simulink model "attempt99999"  (R2026a)
settings: Solver=VariableStepAuto  StopTime=10
values from neighbouring files (symbols this model uses):
  I_x = 3770    [attempt999999.m]
  I_y = 730    [attempt999999.m]
  I_z = 4020    [attempt999999.m]
  omega_0 = 7.272 * 10^-5    (= 7.272e-05)    [attempt999999.m]
settings Model: Creator=syane  LastModifiedBy=syane

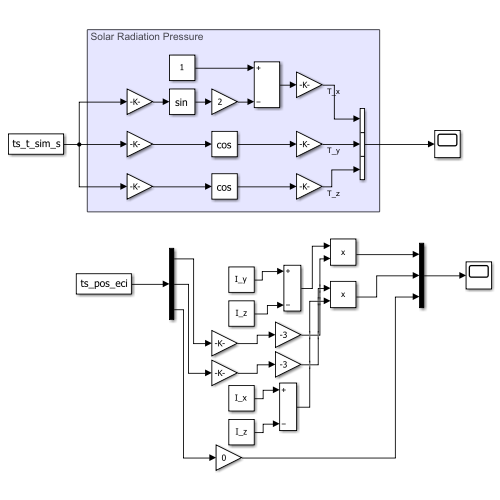
[thumbnail: Simulink's stored preview of the top-level diagram]
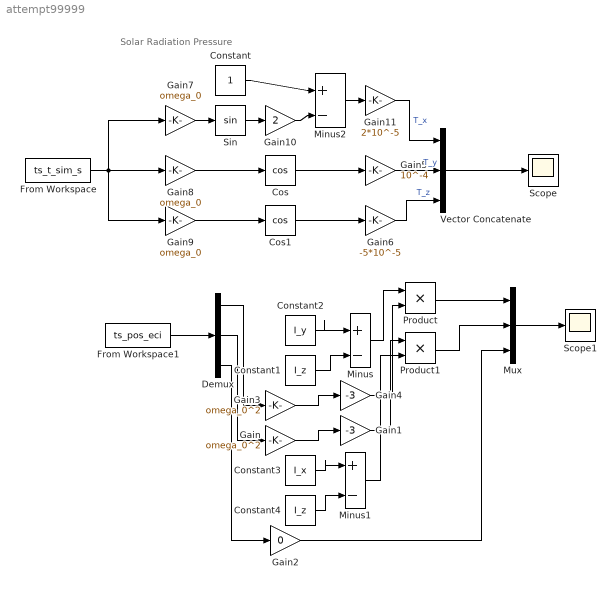
== system attempt99999 ==
  note: Solar Radiation Pressure
  Constant : Constant
  Constant1 : Constant  Value=I_z
  Constant2 : Constant  Value=I_y
  Constant3 : Constant  Value=I_x
  Constant4 : Constant  Value=I_z
  Cos : Trigonometry  Operator=cos
  Cos1 : Trigonometry  Operator=cos
  Demux : Demux  Outputs=3
  From Workspace : FromWorkspace  VariableName=ts_t_sim_s
  From Workspace1 : FromWorkspace  VariableName=ts_pos_eci
  Gain : Gain  Gain=omega_0^2
  Gain1 : Gain  Gain=-3
  Gain10 : Gain  Gain=2
  Gain11 : Gain  Gain=2*10^-5
  Gain2 : Gain  Gain=0
  Gain3 : Gain  Gain=omega_0^2
  Gain4 : Gain  Gain=-3
  Gain5 : Gain  Gain=10^-4
  Gain6 : Gain  Gain=-5*10^-5
  Gain7 : Gain  Gain=omega_0
  Gain8 : Gain  Gain=omega_0
  Gain9 : Gain  Gain=omega_0
  Minus : Sum  Inputs=+|-
  Minus1 : Sum  Inputs=+|-
  Minus2 : Sum  Inputs=+|-
  Mux : Mux  Inputs=3
  Product : Product
  Product1 : Product
  Scope : Scope
      settings: ActiveDisplayYMinimum=-6.875E-5  ActiveDisplayYMaximum=0.00011875000000000001
  Scope1 : Scope
      settings: ActiveDisplayYMinimum=144.59611410559012  ActiveDisplayYMaximum=155.72041159354291
  Sin : Trigonometry
  Vector Concatenate : Concatenate  NumInputs=3
  wires:
  Vector Concatenate/1 -> Scope/1
  Gain/1 -> Gain1/1
  Constant3/1 -> Minus1/1
  Constant4/1 -> Minus1/2
  Demux/3 -> Gain2/1
  Gain3/1 -> Gain4/1
  Demux/2 -> Gain/1
  Demux/1 -> Gain3/1
  Gain4/1 -> Product/2
  Minus/1 -> Product/1
  Product/1 -> Mux/1
  Gain1/1 -> Product1/1
  Minus1/1 -> Product1/2
  Product1/1 -> Mux/2
  Gain2/1 -> Mux/3
  Mux/1 -> Scope1/1
  From Workspace1/1 -> Demux/1
  Constant1/1 -> Minus/2
  Constant2/1 -> Minus/1
  Gain9/1 -> Cos1/1
  Cos1/1 -> Gain6/1
  Gain8/1 -> Cos/1
  Gain5/1 -> Vector Concatenate/2  "T_y"
  Constant/1 -> Minus2/1
  Sin/1 -> Gain10/1
  Gain10/1 -> Minus2/2
  Minus2/1 -> Gain11/1
  Gain7/1 -> Sin/1
  Gain6/1 -> Vector Concatenate/3  "T_z"
  Gain11/1 -> Vector Concatenate/1  "T_x"
  From Workspace/1 -> Gain7/1, Gain9/1, Gain8/1
  Cos/1 -> Gain5/1
